simulink model "Zustandsregelung_mit_I_Regelung_nichtlinear"  (R2021b)
settings: Solver=FixedStepAuto  StartTime=0.0  StopTime=10  FixedStep=1/1e4  RelTol=1e-3
undefined symbols (not defined in the file): C_buck, d, k_LMI_3_Tilde, L_buck, S, T_c, x_Ruhe, y_ref_I_Reg
settings Model: Creator=basti  LastModifiedBy=basti

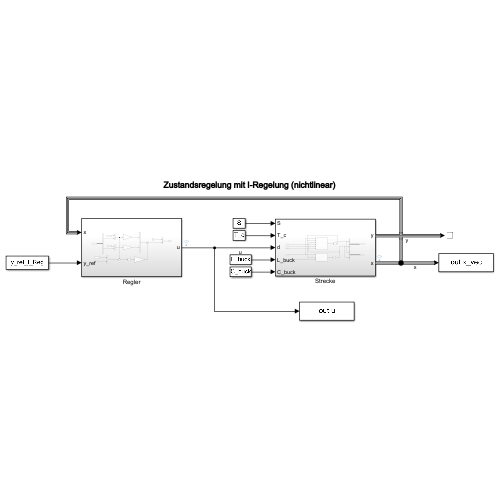
[thumbnail: Simulink's stored preview of the top-level diagram]
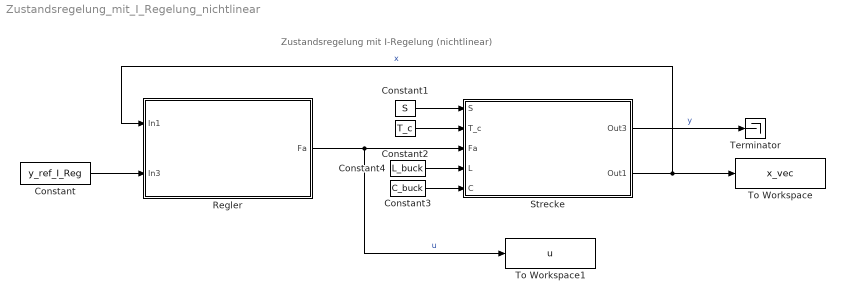
== system Zustandsregelung_mit_I_Regelung_nichtlinear ==
  note: Zustandsregelung mit I-Regelung (nichtlinear)
  Constant : Constant  Value=y_ref_I_Reg
  Constant1 : Constant  Value=S
  Constant2 : Constant  Value=T_c
  Constant3 : Constant  Value=C_buck
  Constant4 : Constant  Value=L_buck
  Regler : Subsystem
  Strecke : Subsystem
  Terminator : Terminator
  To Workspace : ToWorkspace  VariableName=x_vec  SaveFormat=Timeseries  SampleTime=-1
  To Workspace1 : ToWorkspace  VariableName=u  SaveFormat=Timeseries  SampleTime=-1
  wires:
  Constant/1 -> Regler/2(In3)
  Strecke/1(Out3) -> Terminator/1  "y"
  Strecke/2(Out1) -> Regler/1(In1), To Workspace/1  "x"
  Constant4/1 -> Strecke/4(L)
  Constant1/1 -> Strecke/1(S)
  Constant2/1 -> Strecke/2(T_c)
  Constant3/1 -> Strecke/5(C)
  Regler/1(Fa) -> To Workspace1/1, Strecke/3(Fa)  "u"

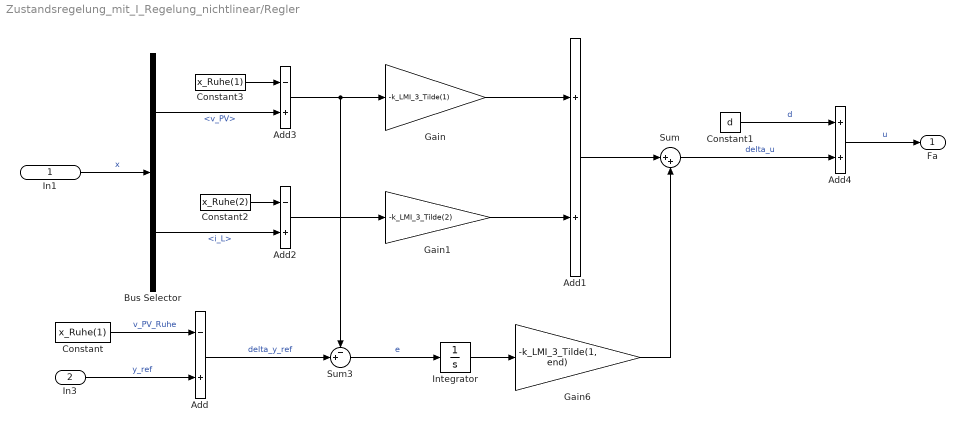
== system Zustandsregelung_mit_I_Regelung_nichtlinear/Regler ==
  In1 : Inport
  In3 : Inport  Port=2
  Add : Sum  Inputs=-+
  Add1 : Sum
  Add2 : Sum  Inputs=-+
  Add3 : Sum  Inputs=-+
  Add4 : Sum
  Bus Selector : BusSelector  OutputSignals=v_PV,i_L
  Constant : Constant  Value=x_Ruhe(1)
  Constant1 : Constant  Value=d
  Constant2 : Constant  Value=x_Ruhe(2)
  Constant3 : Constant  Value=x_Ruhe(1)
  Gain : Gain  Gain=-k_LMI_3_Tilde(1)
  Gain1 : Gain  Gain=-k_LMI_3_Tilde(2)
  Gain6 : Gain  Gain=-k_LMI_3_Tilde(1, end)
  Integrator : Integrator
  Sum : Sum  Inputs=|++
  Sum3 : Sum  Inputs=-+|
  Fa : Outport
  wires:
  Gain6/1 -> Sum/2
  In3/1 -> Add/2  "y_ref"
  Sum/1 -> Add4/2  "delta_u"
  Integrator/1 -> Gain6/1
  Sum3/1 -> Integrator/1  "e"
  Add1/1 -> Sum/1
  Gain/1 -> Add1/1
  In1/1 -> Bus Selector/1  "x"
  Bus Selector/1 -> Add3/2  "<v_PV>"
  Gain1/1 -> Add1/2
  Bus Selector/2 -> Add2/2  "<i_L>"
  Constant/1 -> Add/1  "v_PV_Ruhe"
  Constant2/1 -> Add2/1
  Constant3/1 -> Add3/1
  Add3/1 -> Gain/1, Sum3/1
  Add2/1 -> Gain1/1
  Constant1/1 -> Add4/1  "d"
  Add4/1 -> Fa/1  "u"
  Add/1 -> Sum3/2  "delta_y_ref"

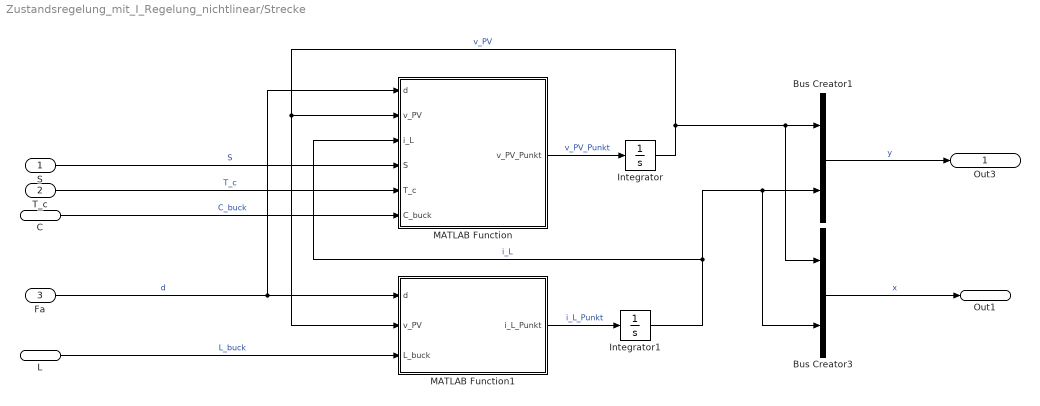
== system Zustandsregelung_mit_I_Regelung_nichtlinear/Strecke ==
  S : Inport
  T_c : Inport  Port=2
  Fa : Inport  Port=3
  L : Inport  Port=4
  C : Inport  Port=5
  Bus Creator1 : BusCreator  Inputs=2
  Bus Creator3 : BusCreator  Inputs=2
  Integrator : Integrator  InitialCondition=x_Ruhe(1)
  Integrator1 : Integrator  InitialCondition=x_Ruhe(2)
  MATLAB Function : MATLAB Function  TreatAsAtomicUnit=on
  MATLAB Function1 : MATLAB Function  TreatAsAtomicUnit=on
  Out3 : Outport
  Out1 : Outport  Port=2
  wires:
  Fa/1 -> MATLAB Function1/1(d), MATLAB Function/1(d)  "d"
  Integrator1/1 -> MATLAB Function/3(i_L), Bus Creator1/2, Bus Creator3/2  "i_L"
  Bus Creator1/1 -> Out3/1  "y"
  T_c/1 -> MATLAB Function/5(T_c)  "T_c"
  MATLAB Function1/1(i_L_Punkt) -> Integrator1/1  "i_L_Punkt"
  C/1 -> MATLAB Function/6(C_buck)  "C_buck"
  L/1 -> MATLAB Function1/3(L_buck)  "L_buck"
  MATLAB Function/1(v_PV_Punkt) -> Integrator/1  "v_PV_Punkt"
  Integrator/1 -> Bus Creator1/1, Bus Creator3/1, MATLAB Function/2(v_PV), MATLAB Function1/2(v_PV)  "v_PV"
  S/1 -> MATLAB Function/4(S)  "S"
  Bus Creator3/1 -> Out1/1  "x"

== matlab function Zustandsregelung_mit_I_Regelung_nichtlinear/Strecke/MATLAB Function1 ==
  data: d input; i_L_Punkt output; v_PV input; L_buck input
function i_L_Punkt = fcn(d, v_PV, L_buck)
    % Konstanten
    c = Konstanten();

    % Berechnung
    i_L_Punkt = 1/L_buck * v_PV * d - 1/L_buck * c.v_DC;

== matlab function Zustandsregelung_mit_I_Regelung_nichtlinear/Strecke/MATLAB Function ==
  data: d input; v_PV_Punkt output; v_PV input; i_L input; S input; T_c input; C_buck input
% Eingänge

% Ausgänge

function v_PV_Punkt = fcn(d, v_PV, i_L, S, T_c, C_buck)
    % Konstanten
    c = Konstanten();

    % Berechnung
    v_oc = @(T_c) c.v_oc_STC * (1 + c.beta_T * (T_c - c.T_c_STC));                                      % für Modul
    i_ph = @(S, T_c) (S/c.S_STC) * c.i_ph_sc_STC * (1 + c.alpha_T * (T_c - c.T_c_STC));                 % für Modul
    i_s = @(S, T_c) (i_ph(S, T_c) - (v_oc(T_c)/c.R_h))/(exp(v_oc(T_c)/(c.A_n * c.v_T_STC)) - 1);        % für Modul
    i_d = @(x1, S, T_c) i_s(S, T_c) * (exp(x1/(c.N_s*c.v_T_STC * c.A_n)) - 1);                          % für Modul

    i_pv = @(x1, S, T_c) c.N_p * (i_ph(S, T_c) - i_d(x1, S, T_c) - x1/(c.N_s * c.R_h));

    v_PV_Punkt = 1/C_buck * i_pv(v_PV, S, T_c) - 1/C_buck * i_L * d;
